simulink model "MotionController"  (Simulink 7.5)
settings: Solver=FixedStepDiscrete  StartTime=0.0  StopTime=inf  FixedStep=0.02  RelTol=1e-3
values from neighbouring files (symbols this model uses):
  Depth_Kd = 0    [controlConstants.m]
  Depth_Ki = 0    [controlConstants.m]
  Depth_Kp = 1    [controlConstants.m]
  IMU_YawRate_Kd = 0    [controlConstants.m]
  IMU_YawRate_Ki = 0    [controlConstants.m]
  IMU_YawRate_Kp = 1    [controlConstants.m]
  IMU_YVel_Kd = 0    [controlConstants.m]
  IMU_YVel_Ki = 0    [controlConstants.m]
  IMU_YVel_Kp = 1    [controlConstants.m]
undefined symbols (not defined in the file or in its folder): DiscIntNeverNeededParam, Heading_Kd, Heading_Ki, Heading_Kp
libraries: simulink x7
settings Model: Creator=auvt  LastModifiedBy=auvt  ParamWorkspaceSource=ReferencedWorkspace  TunableVars=Depth_Kd,Depth_Ki,Depth_Kp,Heading_Kd,Heading_Ki,Heading_Kp,IMU_YVel_Kd,IMU_YVel_Ki,IMU_YVel_Kp,IMU_YawRate_Kd,IMU_YawRate_Ki,IMU_YawRate_Kp  TunableVarsStorageClass=Auto,Auto,Auto,Auto,Auto,Auto,Auto,Auto,Auto,Auto,Auto,Auto  TunableVarsTypeQualifier=,,,,,,,,,,,
settings OptimizationCC: InlineParams=on  OptimizeModelRefInitCode=on  LifeSpan=1
settings RTWCC: SystemTargetFile=ert.tlc  GenCodeOnly=on  TemplateMakefile=ert_default_tmf  Description=Real-Time Workshop Embedded Coder  ProcessScript=ert_make_rtw_hook  TargetLang=C++
settings CodeAppCC: IgnoreCustomStorageClasses=off
settings ERTTargetCC: MultiwordLength=2048  GenerateSampleERTMain=on  IncludeMdlTerminateFcn=off  InlinedParameterPlacement=NonHierarchical  ERTCustomFileTemplate=example_file_process.tlc  ConvertIfToSwitch=off

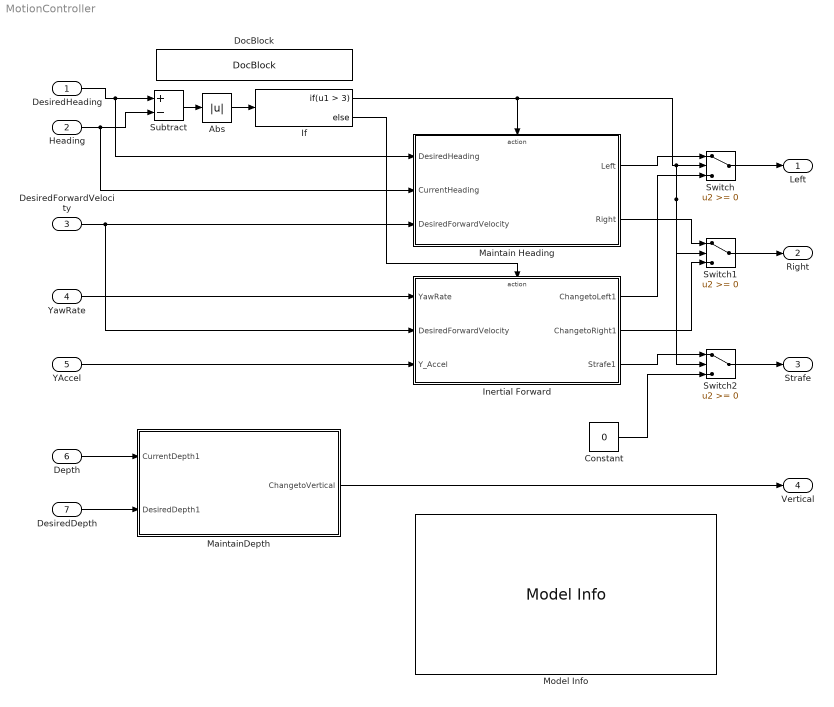
== system MotionController ==
  DesiredHeading : Inport  OutDataType=fixdt(1, 16)  OutScaling=2^0
  Heading : Inport  Port=2  OutDataType=fixdt(1, 16)  OutScaling=2^0
  DesiredForwardVelocity : Inport  Port=3  OutDataType=fixdt(1, 16)  OutScaling=2^0
  YawRate : Inport  Port=4  OutDataType=fixdt(1, 16)  OutScaling=2^0
  YAccel : Inport  Port=5  OutDataType=fixdt(1, 16)  OutScaling=2^0
  Depth : Inport  Port=6  OutDataType=fixdt(1, 16)  OutScaling=2^0
  DesiredDepth : Inport  Port=7  OutDataType=fixdt(1, 16)  OutScaling=2^0
  Abs : Abs  OutDataType=fixdt(1, 16)  OutScaling=2^0
  Constant : Constant  Value=0  OutDataType=fixdt(1, 16)  OutScaling=2^0
  DocBlock : simulink/Model-Wide Utilities/DocBlock  SystemSampleTime=-1  DocumentType=Text
  If : If  IfExpression=u1 > 3
  "Inertial Forward " : Subsystem
      settings: UndoDeleteFcn=Stateflow.SLINSF.SimulinkMan.restorePreDeleteFcn  PreDeleteFcn=Stateflow.SLINSF.SimulinkMan.removePreDeleteFcn
  Maintain Heading : Subsystem  TreatAsAtomicUnit=on
  "MaintainDepth " : Subsystem
      settings: UndoDeleteFcn=Stateflow.SLINSF.SimulinkMan.restorePreDeleteFcn  PreDeleteFcn=Stateflow.SLINSF.SimulinkMan.removePreDeleteFcn
  Model Info : simulink/Model-Wide Utilities/Model Info  SystemSampleTime=-1  InitialBlockCM=None  BlockCM=None  Frame=on  DisplayStringWithTags=|  HorizontalTextAlignment=Left  LeftAlignmentValue=0.02  SourceBlockDiagram=MotionController  TagMaxNumber=20
      | This Model directly controls the
      |  thrusters by using several controllers. 
      |  The controllers are based on current
      |  state information (heading, depth, etc.)
      |  as well as desired state info.
      | 
      | %<LastModifiedBy>
      | %<LastModificationDate>
  Subtract : Sum  Inputs=+-  OutDataType=fixdt(1, 16)  OutScaling=2^-10
  Switch : Switch  OutDataType=fixdt(1, 16)  OutScaling=2^0
  Switch1 : Switch  OutDataType=fixdt(1, 16)  OutScaling=2^0
  Switch2 : Switch  OutDataType=fixdt(1, 16)  OutScaling=2^0
  Left : Outport  OutDataType=fixdt(1, 16)  OutScaling=2^0
  Right : Outport  Port=2  OutDataType=fixdt(1, 16)  OutScaling=2^0
  Strafe : Outport  Port=3  OutDataType=fixdt(1, 16)  OutScaling=2^0
  Vertical : Outport  Port=4  OutDataType=fixdt(1, 16)  OutScaling=2^0
  wires:
  If/1 -> Maintain Heading/Action, Switch/2, Switch1/2, Switch2/2
  If/2 -> "Inertial Forward "/Action
  Depth/1 -> "MaintainDepth "/1(CurrentDepth1)
  DesiredDepth/1 -> "MaintainDepth "/2(DesiredDepth1)
  DesiredHeading/1 -> Subtract/1, Maintain Heading/1(DesiredHeading)
  Subtract/1 -> Abs/1
  Abs/1 -> If/1
  Heading/1 -> Subtract/2, Maintain Heading/2(CurrentHeading)
  DesiredForwardVelocity/1 -> Maintain Heading/3(DesiredForwardVelocity), "Inertial Forward "/2(DesiredForwardVelocity)
  YawRate/1 -> "Inertial Forward "/1(YawRate)
  YAccel/1 -> "Inertial Forward "/3(Y_Accel)
  Maintain Heading/1(Left) -> Switch/1
  "Inertial Forward "/1(ChangetoLeft1) -> Switch/3
  Switch/1 -> Left/1
  Maintain Heading/2(Right) -> Switch1/1
  "Inertial Forward "/2(ChangetoRight1) -> Switch1/3
  Constant/1 -> Switch2/3
  "Inertial Forward "/3(Strafe1) -> Switch2/1
  Switch1/1 -> Right/1
  Switch2/1 -> Strafe/1
  "MaintainDepth "/1(ChangetoVertical) -> Vertical/1

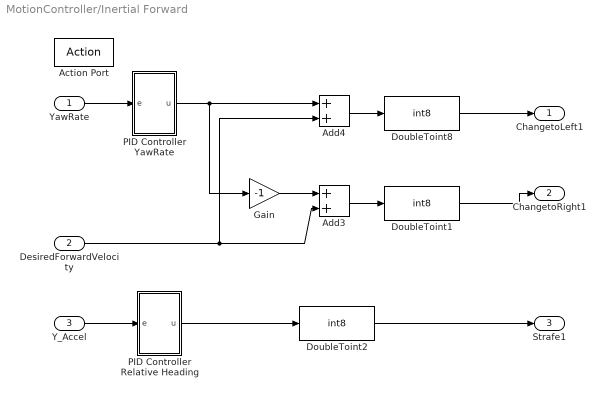
== system MotionController/Inertial Forward  ==
  YawRate : Inport
  DesiredForwardVelocity : Inport  Port=2  OutDataType=fixdt(1, 16)  OutScaling=2^0
  Y_Accel : Inport  Port=3
  Action Port : ActionPort  ActionType=else
  Add3 : Sum  OutDataType=fixdt(1, 16)  OutScaling=2^-10
  Add4 : Sum  OutDataType=fixdt(1, 16)  OutScaling=2^-10
  DoubleToint1 : DataTypeConversion  OutDataTypeMode=int8  OutDataType=fixdt(1, 16)  OutScaling=2^0  OutDataTypeStr=int8  SaturateOnIntegerOverflow=on
  DoubleToint2 : DataTypeConversion  OutDataTypeMode=int8  OutDataType=fixdt(1, 16)  OutScaling=2^0  OutDataTypeStr=int8  SaturateOnIntegerOverflow=on
  DoubleToint8 : DataTypeConversion  OutDataTypeMode=int8  OutDataType=fixdt(1, 16)  OutScaling=2^0  OutDataTypeStr=int8  SaturateOnIntegerOverflow=on
  Gain : Gain  Gain=-1  ParameterDataType=fixdt(1, 16)  ParameterScaling=2^0  OutDataType=fixdt(1, 16)  OutScaling=2^0
  PID Controller Relative Heading : Subsystem  Description=PID
  PID Controller YawRate : Subsystem  Description=PID
  ChangetoLeft1 : Outport  OutDataType=fixdt(1, 16)  OutScaling=2^0
  ChangetoRight1 : Outport  Port=2  OutDataType=fixdt(1, 16)  OutScaling=2^0
  Strafe1 : Outport  Port=3  OutDataType=fixdt(1, 16)  OutScaling=2^0
  wires:
  DoubleToint2/1 -> Strafe1/1
  PID Controller Relative Heading/1(u) -> DoubleToint2/1
  Y_Accel/1 -> PID Controller Relative Heading/1(e)
  DoubleToint1/1 -> ChangetoRight1/1
  DoubleToint8/1 -> ChangetoLeft1/1
  Gain/1 -> Add3/1
  YawRate/1 -> PID Controller YawRate/1(e)
  DesiredForwardVelocity/1 -> Add3/2, Add4/2
  Add3/1 -> DoubleToint1/1
  Add4/1 -> DoubleToint8/1
  PID Controller YawRate/1(u) -> Gain/1, Add4/1

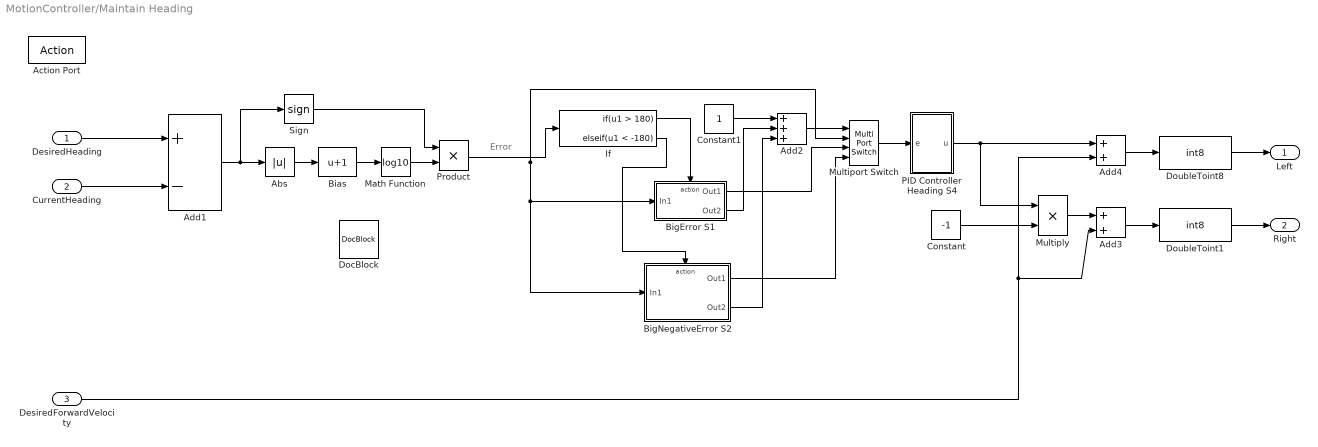
== system MotionController/Maintain Heading ==
  note: Error
  DesiredHeading : Inport  PortDimensions=1  OutDataType=fixdt(1, 16)  OutScaling=2^0
  CurrentHeading : Inport  Port=2  PortDimensions=1  OutDataType=fixdt(1, 16)  OutScaling=2^0
  DesiredForwardVelocity : Inport  Port=3  OutDataType=fixdt(1, 16)  OutScaling=2^0
  Action Port : ActionPort  ActionType=then
  Abs : Abs  OutDataType=fixdt(1, 16)  OutScaling=2^0
  Add1 : Sum  Inputs=+-  AccumDataTypeStr=double  OutDataType=fixdt(1, 16)  OutScaling=2^-10
  Add2 : Sum  Inputs=+++  OutDataType=fixdt(1, 16)  OutScaling=2^-10
  Add3 : Sum  OutDataType=fixdt(1, 16)  OutScaling=2^-10
  Add4 : Sum  OutDataType=fixdt(1, 16)  OutScaling=2^-10
  Bias : Bias  Bias=1
  BigError S1 : Subsystem  TreatAsAtomicUnit=on
  BigNegativeError S2 : Subsystem  TreatAsAtomicUnit=on
  Constant : Constant  Value=-1  OutDataTypeMode=int8  OutDataType=fixdt(1, 16)  OutScaling=2^0  OutDataTypeStr=int8  SampleTime=-1
  Constant1 : Constant  OutDataType=fixdt(1, 16)  OutScaling=2^0  SampleTime=-1
  DocBlock : simulink/Model-Wide Utilities/DocBlock  SystemSampleTime=-1  DocumentType=Text
  DoubleToint1 : DataTypeConversion  OutDataTypeMode=int8  OutDataType=fixdt(1, 16)  OutScaling=2^0  OutDataTypeStr=int8  SaturateOnIntegerOverflow=on
  DoubleToint8 : DataTypeConversion  OutDataTypeMode=int8  OutDataType=fixdt(1, 16)  OutScaling=2^0  OutDataTypeStr=int8  SaturateOnIntegerOverflow=on
  If : If  IfExpression=u1 > 180  ElseIfExpressions=u1 < -180  ShowElse=off
  Math Function : Math  Operator=log10  OutDataType=fixdt(1, 16)  OutScaling=2^0  SaturateOnIntegerOverflow=on
  Multiply : Product  Inputs=**  OutDataTypeMode=int8  OutDataType=fixdt(1, 16)  OutScaling=2^-10  OutDataTypeStr=int8
  Multiport Switch : MultiPortSwitch  zeroidx=off  OutDataType=fixdt(1, 16)  OutScaling=2^0
  PID Controller Heading S4 : Subsystem  Description=PID
  Product : Product  OutDataType=fixdt(1, 16)  OutScaling=2^0  RndMeth=Zero
  Sign : Signum
  Left : Outport  OutDataType=fixdt(1, 16)  OutScaling=2^0
  Right : Outport  Port=2  OutDataType=fixdt(1, 16)  OutScaling=2^0
  wires:
  DesiredHeading/1 -> Add1/1
  Constant/1 -> Multiply/2
  Add1/1 -> Abs/1, Sign/1
  If/1 -> BigError S1/Action
  If/2 -> BigNegativeError S2/Action
  BigError S1/1(Out1) -> Multiport Switch/3
  BigNegativeError S2/1(Out1) -> Multiport Switch/4
  Multiport Switch/1 -> PID Controller Heading S4/1(e)
  Constant1/1 -> Add2/1
  BigError S1/2(Out2) -> Add2/2
  BigNegativeError S2/2(Out2) -> Add2/3
  Add2/1 -> Multiport Switch/1
  CurrentHeading/1 -> Add1/2
  Multiply/1 -> Add3/1
  DesiredForwardVelocity/1 -> Add3/2, Add4/2
  Add3/1 -> DoubleToint1/1
  DoubleToint1/1 -> Right/1
  Add4/1 -> DoubleToint8/1
  DoubleToint8/1 -> Left/1
  PID Controller Heading S4/1(u) -> Add4/1, Multiply/1
  Bias/1 -> Math Function/1
  Abs/1 -> Bias/1
  Sign/1 -> Product/1
  Math Function/1 -> Product/2
  Product/1 -> If/1, BigError S1/1(In1), BigNegativeError S2/1(In1), Multiport Switch/2

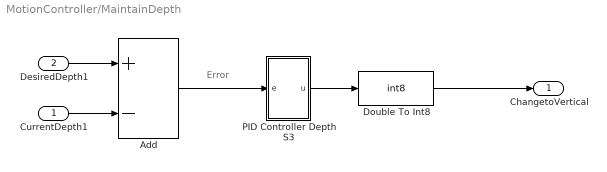
== system MotionController/MaintainDepth  ==
  note: Error
  CurrentDepth1 : Inport  DataType=single  OutDataType=fixdt(1, 16)  OutScaling=2^0  OutDataTypeStr=single
  DesiredDepth1 : Inport  Port=2  DataType=single  OutDataType=fixdt(1, 16)  OutScaling=2^0  OutDataTypeStr=single
  Add : Sum  Inputs=+-  OutDataTypeMode=double  OutDataType=fixdt(1, 16)  OutScaling=2^-10  OutDataTypeStr=double
  Double To Int8 : DataTypeConversion  OutDataTypeMode=int8  OutDataType=fixdt(1, 16)  OutScaling=2^0  OutDataTypeStr=int8  SaturateOnIntegerOverflow=on
  PID Controller Depth S3 : Subsystem  Description=PID
  ChangetoVertical : Outport  DataType=int8  OutDataType=fixdt(1, 16)  OutScaling=2^0  OutDataTypeStr=int8
  wires:
  Add/1 -> PID Controller Depth S3/1(e)
  PID Controller Depth S3/1(u) -> Double To Int8/1
  Double To Int8/1 -> ChangetoVertical/1
  CurrentDepth1/1 -> Add/2
  DesiredDepth1/1 -> Add/1

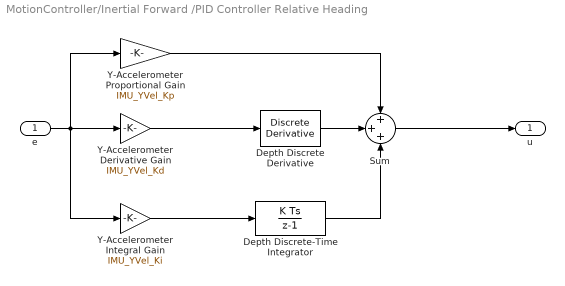
== system MotionController/Inertial Forward /PID Controller Relative Heading ==
  e : Inport
  Depth Discrete Derivative : simulink/Discrete/Discrete Derivative  SystemSampleTime=-1  gainval=1  ICPrevScaledInput=0.0  OutMin=[]  OutMax=[]  OutDataType=fixdt(1, 16)  OutScaling=2^-10  DoSatur=on
  Depth Discrete-Time Integrator : DiscreteIntegrator  gainval=1  SampleTime=-1  OutDataType=fixdt(1, 16)  OutScaling=2^0  LimitOutput=on  UpperSaturationLimit=10  LowerSaturationLimit=-10  ICPrevOutput=DiscIntNeverNeededParam  ICPrevScaledInput=DiscIntNeverNeededParam
  Sum : Sum  Inputs=+++  OutDataType=sfix(16)  OutScaling=2^0  SaturateOnIntegerOverflow=on  InputSameDT=on  OutDataTypeStr=Inherit: Same as first input
  Y-Accelerometer Derivative Gain : Gain  Gain=IMU_YVel_Kd  ParameterDataType=fixdt(1, 16)  ParameterScaling=2^0  OutDataType=fixdt(1, 16)  OutScaling=2^0
  Y-Accelerometer Integral Gain : Gain  Gain=IMU_YVel_Ki  ParameterDataType=fixdt(1, 16)  ParameterScaling=2^0  OutDataType=fixdt(1, 16)  OutScaling=2^0
  Y-Accelerometer Proportional Gain : Gain  Gain=IMU_YVel_Kp  ParameterDataType=fixdt(1, 16)  ParameterScaling=2^0  OutDataType=fixdt(1, 16)  OutScaling=2^0
  u : Outport
  wires:
  e/1 -> Y-Accelerometer Proportional Gain/1, Y-Accelerometer Derivative Gain/1, Y-Accelerometer Integral Gain/1
  Depth Discrete-Time Integrator/1 -> Sum/3
  Y-Accelerometer Proportional Gain/1 -> Sum/1
  Sum/1 -> u/1
  Depth Discrete Derivative/1 -> Sum/2
  Y-Accelerometer Derivative Gain/1 -> Depth Discrete Derivative/1
  Y-Accelerometer Integral Gain/1 -> Depth Discrete-Time Integrator/1

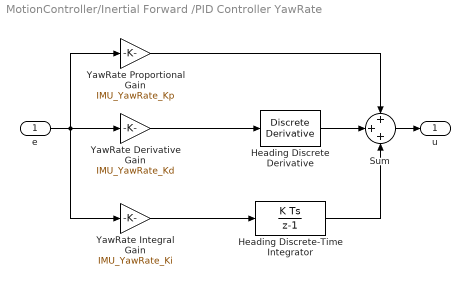
== system MotionController/Inertial Forward /PID Controller YawRate ==
  e : Inport
  Heading Discrete Derivative : simulink/Discrete/Discrete Derivative  SystemSampleTime=-1  gainval=1  ICPrevScaledInput=0.0  OutMin=[]  OutMax=[]  OutDataType=fixdt(1, 16)  OutScaling=2^-10  DoSatur=off
  Heading Discrete-Time Integrator : DiscreteIntegrator  gainval=1  SampleTime=-1  OutDataType=fixdt(1, 16)  OutScaling=2^0  LimitOutput=on  UpperSaturationLimit=15  LowerSaturationLimit=-15  ICPrevOutput=DiscIntNeverNeededParam  ICPrevScaledInput=DiscIntNeverNeededParam
  Sum : Sum  Inputs=+++  OutDataType=sfix(16)  OutScaling=2^0  SaturateOnIntegerOverflow=on  InputSameDT=on  OutDataTypeStr=Inherit: Same as first input
  YawRate Derivative Gain : Gain  Gain=IMU_YawRate_Kd  ParameterDataType=fixdt(1, 16)  ParameterScaling=2^0  OutDataType=fixdt(1, 16)  OutScaling=2^0
  YawRate Integral Gain : Gain  Gain=IMU_YawRate_Ki  ParameterDataType=fixdt(1, 16)  ParameterScaling=2^0  OutDataType=fixdt(1, 16)  OutScaling=2^0
  YawRate Proportional Gain : Gain  Gain=IMU_YawRate_Kp  ParameterDataType=fixdt(1, 16)  ParameterScaling=2^0  OutDataType=fixdt(1, 16)  OutScaling=2^0
  u : Outport
  wires:
  e/1 -> YawRate Proportional Gain/1, YawRate Derivative Gain/1, YawRate Integral Gain/1
  Heading Discrete-Time Integrator/1 -> Sum/3
  YawRate Proportional Gain/1 -> Sum/1
  Sum/1 -> u/1
  Heading Discrete Derivative/1 -> Sum/2
  YawRate Derivative Gain/1 -> Heading Discrete Derivative/1
  YawRate Integral Gain/1 -> Heading Discrete-Time Integrator/1

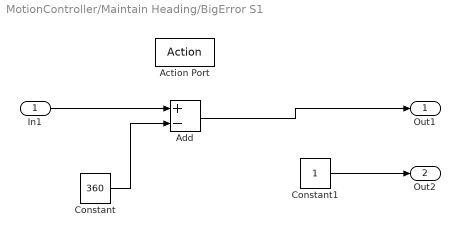
== system MotionController/Maintain Heading/BigError S1 ==
  In1 : Inport  OutDataType=fixdt(1, 16)  OutScaling=2^0
  Action Port : ActionPort  PropagateVarSize=During execution  ActionType=then
  Add : Sum  Inputs=+-  OutDataType=fixdt(1, 16)  OutScaling=2^-10
  Constant : Constant  Value=360  OutDataType=fixdt(1, 16)  OutScaling=2^0  SampleTime=-1
  Constant1 : Constant  OutDataType=fixdt(1, 16)  OutScaling=2^0  SampleTime=-1
  Out1 : Outport  OutDataType=fixdt(1, 16)  OutScaling=2^0
  Out2 : Outport  Port=2  OutDataType=fixdt(1, 16)  OutScaling=2^0  OutputWhenDisabled=reset  InitialOutput=[0]
  wires:
  In1/1 -> Add/1
  Constant/1 -> Add/2
  Add/1 -> Out1/1
  Constant1/1 -> Out2/1

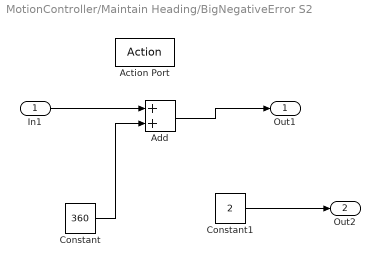
== system MotionController/Maintain Heading/BigNegativeError S2 ==
  In1 : Inport  OutDataType=fixdt(1, 16)  OutScaling=2^0
  Action Port : ActionPort  PropagateVarSize=During execution  ActionType=elseif
  Add : Sum  OutDataType=fixdt(1, 16)  OutScaling=2^-10
  Constant : Constant  Value=360  OutDataType=fixdt(1, 16)  OutScaling=2^0  SampleTime=-1
  Constant1 : Constant  Value=2  OutDataType=fixdt(1, 16)  OutScaling=2^0  SampleTime=-1
  Out1 : Outport  OutDataType=fixdt(1, 16)  OutScaling=2^0
  Out2 : Outport  Port=2  OutDataType=fixdt(1, 16)  OutScaling=2^0  OutputWhenDisabled=reset  InitialOutput=[0]
  wires:
  In1/1 -> Add/1
  Constant/1 -> Add/2
  Add/1 -> Out1/1
  Constant1/1 -> Out2/1

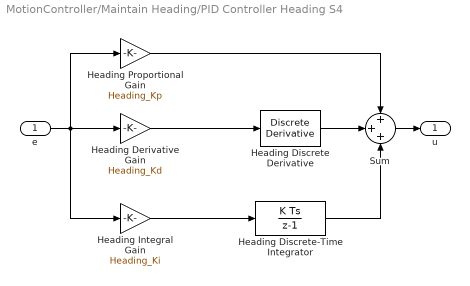
== system MotionController/Maintain Heading/PID Controller Heading S4 ==
  e : Inport
  Heading Derivative Gain : Gain  Gain=Heading_Kd  ParameterDataType=fixdt(1, 16)  ParameterScaling=2^0  OutDataType=fixdt(1, 16)  OutScaling=2^0
  Heading Discrete Derivative : simulink/Discrete/Discrete Derivative  SystemSampleTime=-1  gainval=1  ICPrevScaledInput=0.0  OutMin=[]  OutMax=[]  OutDataType=fixdt(1, 16)  OutScaling=2^-10  DoSatur=off
  Heading Discrete-Time Integrator : DiscreteIntegrator  gainval=1  SampleTime=-1  OutDataType=fixdt(1, 16)  OutScaling=2^0  LimitOutput=on  UpperSaturationLimit=15  LowerSaturationLimit=-15  ICPrevOutput=DiscIntNeverNeededParam  ICPrevScaledInput=DiscIntNeverNeededParam
  Heading Integral Gain : Gain  Gain=Heading_Ki  ParameterDataType=fixdt(1, 16)  ParameterScaling=2^0  OutDataType=fixdt(1, 16)  OutScaling=2^0
  Heading Proportional Gain : Gain  Gain=Heading_Kp  ParameterDataType=fixdt(1, 16)  ParameterScaling=2^0  OutDataType=fixdt(1, 16)  OutScaling=2^0
  Sum : Sum  Inputs=+++  OutDataType=sfix(16)  OutScaling=2^0  SaturateOnIntegerOverflow=on  InputSameDT=on  OutDataTypeStr=Inherit: Same as first input
  u : Outport
  wires:
  e/1 -> Heading Proportional Gain/1, Heading Derivative Gain/1, Heading Integral Gain/1
  Heading Discrete-Time Integrator/1 -> Sum/3
  Heading Proportional Gain/1 -> Sum/1
  Sum/1 -> u/1
  Heading Discrete Derivative/1 -> Sum/2
  Heading Derivative Gain/1 -> Heading Discrete Derivative/1
  Heading Integral Gain/1 -> Heading Discrete-Time Integrator/1

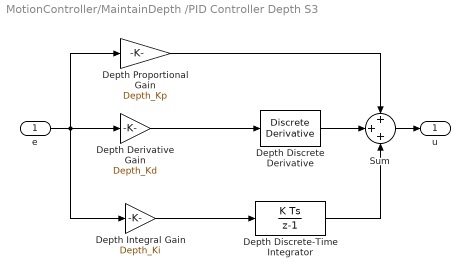
== system MotionController/MaintainDepth /PID Controller Depth S3 ==
  e : Inport
  Depth Derivative Gain : Gain  Gain=Depth_Kd  ParameterDataType=fixdt(1, 16)  ParameterScaling=2^0  OutDataType=fixdt(1, 16)  OutScaling=2^0
  Depth Discrete Derivative : simulink/Discrete/Discrete Derivative  SystemSampleTime=-1  gainval=1  ICPrevScaledInput=0.0  OutMin=[]  OutMax=[]  OutDataType=fixdt(1, 16)  OutScaling=2^-10  DoSatur=on
  Depth Discrete-Time Integrator : DiscreteIntegrator  gainval=1  SampleTime=-1  OutDataType=fixdt(1, 16)  OutScaling=2^0  LimitOutput=on  UpperSaturationLimit=10  LowerSaturationLimit=-10  ICPrevOutput=DiscIntNeverNeededParam  ICPrevScaledInput=DiscIntNeverNeededParam
  Depth Integral Gain : Gain  Gain=Depth_Ki  ParameterDataType=fixdt(1, 16)  ParameterScaling=2^0  OutDataType=fixdt(1, 16)  OutScaling=2^0
  Depth Proportional Gain : Gain  Gain=Depth_Kp  ParameterDataType=fixdt(1, 16)  ParameterScaling=2^0  OutDataType=fixdt(1, 16)  OutScaling=2^0
  Sum : Sum  Inputs=+++  OutDataType=sfix(16)  OutScaling=2^0  SaturateOnIntegerOverflow=on  InputSameDT=on  OutDataTypeStr=Inherit: Same as first input
  u : Outport
  wires:
  e/1 -> Depth Proportional Gain/1, Depth Derivative Gain/1, Depth Integral Gain/1
  Depth Discrete-Time Integrator/1 -> Sum/3
  Depth Proportional Gain/1 -> Sum/1
  Sum/1 -> u/1
  Depth Discrete Derivative/1 -> Sum/2
  Depth Derivative Gain/1 -> Depth Discrete Derivative/1
  Depth Integral Gain/1 -> Depth Discrete-Time Integrator/1
